simulink model "Intergration_simu"  (R2018b)
settings: Solver=FixedStepDiscrete  StartTime=0.0  StopTime=14  FixedStep=0.005  RelTol=1e-3
PostLoadFcn:
  | if any(exist('dsrtsu_mdlpostloadfcn', 'file') ~= 0), dsrtsu_mdlpostloadfcn('Execute', bdroot); end
values from neighbouring files (symbols this model uses):
  P_x165_On = 1.0    [CAN_Tx.sldd]
  P_x242_On = 1.0    [CAN_Tx.sldd]
  P_x246_On = 1.0    [CAN_Tx.sldd]
libraries: rtican x112, simulink x59
(part 25 of 31)

== system Intergration_simu/Radar410_RX/x80 ==
  Bus Creator1 : BusCreator  Inputs=11
  FRS_Status : rtican/RTICAN Receive (RX)   Reserved1=[]  Reserved2=[]  Reserved3=[]  Reserved4=[]  SfcnMessage=[]  Msg_Struct=[]  BoardTypeNo=[]  BoardNo=[]  ChannelNo=[]  Parameters=[]  DialogFcn=[]  UnitName=[]  Revision=[]  UnitValues=[]  DSProperties=struct('RTI',struct('Version',uint32(5),'BlockType',struct('isSLSource',uint8(1),'isSLSink',uint8(1),'isHWSource',uint8(0),'isHWSink',uint8(0),'isSetup',uint8(0),'isInline',uint8(1),'isNonInline',uint8(0),'isInterrupt',uint8(0),'isChannelwise',uint8(0)),'IOBoardType','RTICAN','UnitType','MESSAGE','Identifier','RX','DialogType','MSVC','BlockSet','RTICAN','SlaveProcessor','CAN'))  RTIBlockInterface=struct('OutputPortsWidth',int32([1 1 1 1 1 1 1 1 1 1 1 1 1 1]),'OutputPortsActive',ones(1,14),'OutputPortsName',{{'FRS_Msg_CheckSum','FRS_Msg_AliveCounter','FRS_Status_MisAlign','FRS_Status_HWErr','FRS_Status_BlkProg','FRS_Fail','FRS_MeasEnabled','FRS_Host_Yaw','FRS_HostSpeed','FRS_TimeStamp','FRS_Latency',['RX status'],['RX time'],['RX delta time']}},'OutputPortsDataType',{{'SS_DOUBLE','SS_DOUBLE','SS_DOUBLE','SS_DOUBLE','SS_DOUBLE','SS_DOUBLE','SS_DOUBLE','SS_DOUBLE','SS_DOUBLE','SS_DOUBLE','SS_DOUBLE','SS_DOUBLE','SS_DOUBLE','SS_DOUBLE'}},'OutputPortsLabel',{{'FRS_Msg_CheckSum','FRS_Msg_AliveCounter','FRS_Status_MisAlign','FRS_Status_HWErr','FRS_Status_BlkProg','FRS_Fail','FRS_MeasEnabled','FRS_Host_Yaw','FRS_HostSpeed','FRS_TimeStamp','FRS_Latency','','',''}},'OutputPortsLabelMode','ON','InputPortsWidth',int32(0),'InputPortsActive',0,'DialogFcn','rtican_message_interface_gui','BlockDisplay',{{'','center'}},'IconTransparency','on','ParameterTunableNames',{{}},'InitLevel',3,'BlockName',struct('Token',{{'FRS_Status'}}),'SampleTime',{{-1}},'TriggerPort',{{'none'}},'EnablePort',{{'none'}})  RTIBlockParameters="struct('BoardTypeNo',{{1,'OFF',[]}},'BoardNo',{{2,'ON',[1 16]}},'ChannelNo',{{2,'ON',[1 2]}},'Parameters',{{struct('DataFileSupport',struct('DataFileSelectedMaster',1,'DataFileSelectedLocal',1,'DataFileName','c:\\users\\linqi\\desktop\\matlab\\acc\\dbc\\ars410od_privatecan.dbc|','DataFileDate',{{{['24-11月-2020 15:06:17']}}},'SelectedFile','..\\..\\dbc\\ars410od_privatecan.dbc'),'Options',struct('StatusSelected',1,'TimeSelected',1,'DeltaTimeSelected',1,'BytePortSelected',0,'MessageLengthSelected',0,'TriggerPort',struct('Selected',0,'TriggerType',0),'UserCoding',struct('Selected',0,'InterfaceFile','UserDecodingFile','FcnName','UserDecodeFcn','InportSelected',0,'InportWidth',1,'OutportSelected',0,'OutportWidth',1),'EnablePortSelected',0,'SignalOnPortnameSelected',1,'UseRXService',0),'Message',struct('MsgOnBlocknameSelected',1,'MsgName','FRS_Status','MsgIdFormat',0,'MsgId',128,'MsgLength',8,'NumSignals',11,'SampleTime',-1,'Signal',struct('SgnName',{'FRS_Msg_CheckSum','FRS_Msg_AliveCounter','FRS_Status_MisAlign','FRS_Status_HWErr','FRS_Status_BlkProg','FRS_Fail','FRS_MeasEnabled','FRS_Host_Yaw','FRS_HostSpeed','FRS_TimeStamp','FRS_Latency'},'SgnStartBit',{0,8,12,15,16,17,18,19,30,42,58},'SgnLength',{8,4,3,1,1,1,1,11,12,16,6},'SgnType',{0,0,0,0,0,0,0,0,0,0,0},'ModeValue',{-1,-1,-1,-1,-1,-1,-1,-1,-1,-1,-1},'DataType',{0,0,0,0,0,0,0,0,0,0,0},'ByteLayout',{2,2,2,2,2,2,2,2,2,2,2},'Factor',{1,1,1,1,1,1,1,0.1,0.025,1,2},'Offset',{0,0,0,0,0,0,0,-102.4,-20,0,0},'SgnComment',{{['Check sum shall be generated out of each message content. check sum generation logic is TBC.']},{['Alive counter shall be incremented every radar sensor measurement cycle.']},{['This signal indicates radar sensor mis-alignment status.' char(10) '0x00:unknown' char(10) '0x01:calibrated' char(10) '0x02:sensor mis-alignment detected' char(10) '0x03:calibration in progress' char(10) '0x04:uncalibratable' char(10) '0x05-07:  reserved']},{['Flag to indicate if HW is failed or not.' char(10) '0x0:HW is NOT failed' char(10) '0x1:HW is failed']},{['Sensor blockage status indication.' char(10) '0x0: FRS is NOT blocked' char(10) '0x1: FRS is blocked']},{['This signal indicates if radar is working or not.' char(10) '0x0 = FRS radar is NOT working' char(10) '0x1 = FRS radar is working']},{['This signal indicates if the radar sensor is performing measurement or not. (radio-wave emission or not) Since Conti does not have this, it could be setup as the same as FRS_Fail.' char(10) '']},{['Host vehicle yaw rate in deg/s which is used for radar object tracking (calibrated host yaw rate if sensor has calibration capability).' char(10) 'Left turn is defined as FRS_Host_Yaw positive direction.']},{['Host vehicle over-ground speed which is used for radar object tracking (calibrated host velocity if the sensor has calibaration capability).' char(10) 'Forward movement is defined as FRS_HostSpeed positive direction.']},{['Sensor internal time stamp since the last sensor start up. the time stamp shall loop as it overflows.']},{['Radar process latency in ms from radio-wave reflection observation to CAN message transmission for current cycle.']}},'SgnUnit',{'n/a','n/a','n/a','n/a','n/a','','n/a','deg/s','m/s','s','ms'},'Min',{0,0,0,0,0,0,0,-102.4,-20,0,0},'Max',{255,15,7,1,1,1,1,102.3,82.375,65535,126},'SLDataType',{'SS_DOUBLE','SS_DOUBLE','SS_DOUBLE','SS_DOUBLE','SS_DOUBLE','SS_DOUBLE','SS_DOUBLE','SS_DOUBLE','SS_DOUBLE','SS_DOUBLE','SS_DOUBLE'}),'MsgIdNumFormat',0,'MsgComment',{{'FRS_Status'}}),'Version',1.2,'general',struct('isFromLib',0)),'OFF',[]}},'GroupId',{{struct('Group',{{'RTICAN'}},'No',2,'Behavior',{{'NAMECHANGE'}},'BlockType',{{'SINK'}},'NameChangeFlag',0),'OFF',[]}},'SFcnRTICANMessage',{{struct('MsgType','RX','SFcnPortType','Scalar','MsgName','FRS_Status','MsgIdFormat','STD','MsgId',128,'MsgLength',8,'NumSignals',11,'SampleTime',-1,'Signal',struct('SgnName',{'FRS_Msg_CheckSum','FRS_Msg_AliveCounter','FRS_Status_MisAlign','FRS_Status_HWErr','FRS_Status_BlkProg','FRS_Fail','FRS_MeasEnabled','FRS_Host_Yaw','FRS_HostSpeed','FRS_TimeStamp','FRS_Latency'},'SgnStartBit',{0,8,12,15,16,17,18,19,30,42,58},'SgnLength',{8,4,3,1,1,1,1,11,12,16,6},'SgnType',{'standard','standard','standard','standard','standard','standard','standard','standard','standard','standard','standard'},'ModeValue',{-1,-1,-1,-1,-1,-1,-1,-1,-1,-1,-1},'DataType',{['unsigned int'],['unsigned int'],['unsigned int'],['unsigned int'],['unsigned int'],['unsigned int'],['unsigned int'],['unsigned int'],['unsigned int'],['unsigned int'],['unsigned int']},'ByteLayout',{['motorola back.'],['motorola back.'],['motorola back.'],['motorola back.'],['motorola back.'],['motorola back.'],['motorola back.'],['motorola back.'],['motorola back.'],['motorola back.'],['motorola back.']},'Factor',{1,1,1,1,1,1,1,0.1,0.025,1,2},'Offset',{0,0,0,0,0,0,0,-102.4,-20,0,0},'SLDataType',{'SS_DOUBLE','SS_DOUBLE','SS_DOUBLE','SS_DOUBLE','SS_DOUBLE','SS_DOUBLE','SS_DOUBLE','SS_DOUBLE','SS_DOUBLE','SS_DOUBLE','SS_DOUBLE'}),'StatusSelected','yes','TimeSelected','yes','DeltaTimeSelected','yes','BytePortSelected','no','MessageLengthSelected','no','TriggerPort',struct('Selected','no','TriggerType',0),'UserCoding',struct('Selected','no','InterfaceFile','UserDecodingFile','FcnName','UserDecodeFcn','InportSelected','no','InportWidth',1,'OutportSelected','no','OutportWidth',1),'EnablePortSelected','no','UseRXService','no','BoardType','DS1','BoardNo',1,'ControllerNo',1),'OFF',[]}},'TLCFileName',{{'rtican_rx_message','OFF',[]}})"  RTISFcnParameters=struct('SFcnRTICANMessage','struct','TLCFileName','char')  RTIBlockParaDefault=struct('BoardTypeNo',4302,'BoardNo',1,'ChannelNo',1,'Parameters',struct('DataFileSupport',struct('DataFileSelectedMaster',0,'DataFileSelectedLocal',0,'DataFileName','','DataFileDate','','SelectedFile',['<no file selected>']),'Options',struct('StatusSelected',1,'TimeSelected',1,'DeltaTimeSelected',1,'BytePortSelected',0,'MessageLengthSelected',0,'TriggerPort',struct('Selected',0,'TriggerType','rising'),'UserCoding',struct('Selected',0,'InterfaceFile','UserDecodingFile','FcnName','UserDecodeFcn','InportSelected',0,'InportWidth',1,'OutportSelected',0,'OutportWidth',1),'EnablePortSelected',0,'SignalOnPortnameSelected',1,'UseRXService',0),'Message',struct('MsgOnBlocknameSelected',0,'MsgName',['RX Message'],'MsgIdFormat',0,'MsgId',100,'MsgLength',8,'NumSignals',1,'SampleTime',-1,'Signal',struct('SgnName',['RX signal'],'SgnStartBit',0,'SgnLength',8,'SgnType',0,'ModeValue',-1,'DataType',0,'SLDataType','SS_DOUBLE','ByteLayout',0,'Factor',1,'Offset',0,'Min',0,'Max',255,'SgnComment',{{}},'SgnUnit',''),'MsgIdNumFormat',0,'MsgComment',{{''}}),'Version',1.2,'general',struct('isFromLib',1)),'GroupId',struct('Group',{{'RTICAN'}},'No',1,'Behavior',{{'NAMECHANGE'}},'BlockType',{{'SINK'}},'NameChangeFlag',0),'SFcnRTICANMessage',struct('MsgType','RX','MsgName',['RX Message'],'MsgIdFormat','STD','MsgId',100,'MsgLength',8,'NumSignals',1,'SampleTime',-1,'Signal',struct('SgnName',['RX signal'],'SgnStartBit',0,'SgnLength',8,'SgnType','standard','ModeValue',-1,'DataType',['unsigned int'],'ByteLayout',['little endian'],'SLDataType','SS_DOUBLE','Factor',1,'Offset',0),'StatusSelected','yes','TimeSelected','yes','DeltaTimeSelected','yes','BytePortSelected','no','MessageLengthSelected','no','EnablePortSelected','no','UserCoding',struct('Selected','no','InterfaceFile','UserDecodingFile','FcnName','UserDecodeFcn','InportSelected','no','InportWidth',1,'OutportSelected','no','OutportWidth',1),'TriggerPort',struct('Selected','no','TriggerType','rising'),'UseRXService','no','BoardType','DS4302','BoardNo',1,'ControllerNo',1,'SFcnPortType','Scalar'),'TLCFileName','rtican_rx_message')
      settings: AttributesFormatString=Group Id: RTICAN2\n  SourceProductName=dSPACE RTI CAN Blockset
  Terminator : Terminator
  Terminator1 : Terminator
  Terminator2 : Terminator
  Out1 : Outport
  wires:
  FRS_Status/14 -> Terminator2/1
  FRS_Status/13 -> Terminator1/1
  FRS_Status/12 -> Terminator/1
  Bus Creator1/1 -> Out1/1
  FRS_Status/1 -> Bus Creator1/1  "FRS_Msg_CheckSum"
  FRS_Status/2 -> Bus Creator1/2  "FRS_Msg_AliveCounter"
  FRS_Status/3 -> Bus Creator1/3  "FRS_Status_MisAlign"
  FRS_Status/4 -> Bus Creator1/4  "FRS_Status_HWErr"
  FRS_Status/5 -> Bus Creator1/5  "FRS_Status_BlkProg"
  FRS_Status/6 -> Bus Creator1/6  "FRS_Fail"
  FRS_Status/7 -> Bus Creator1/7  "FRS_MeasEnabled"
  FRS_Status/8 -> Bus Creator1/8  "FRS_Host_Yaw"
  FRS_Status/9 -> Bus Creator1/9  "FRS_HostSpeed"
  FRS_Status/10 -> Bus Creator1/10  "FRS_TimeStamp"
  FRS_Status/11 -> Bus Creator1/11  "FRS_Latency"

== system Intergration_simu/TX/Adapter_Tx ==
  VLC_LgtCmd_st : Inport  OutDataTypeStr=Bus: VLC_LGTCMD_ST
  ACC_LgtCtrl_st : Inport  Port=2
  ATS_Po_st : Inport  Port=3
  Bus Selector : BusSelector  OutputSignals=Valid,dx,dy,Type
  Bus Selector1 : BusSelector  OutputSignals=ACCvSet
  Bus Selector4 : BusSelector  OutputSignals=EngineTorqReq,EngineTorqReqSt,ACCState,CDDEnable,CDDAxtar,CDDDriveoffReq,CDDStandstillReq
  calc_0x165 : Subsystem
  calc_0x242 : Subsystem
  calc_0x246 : Subsystem
  calc_0x255 : Subsystem
  x242 : Outport  OutDataTypeStr=Bus: x242
  x165 : Outport  Port=2  OutDataTypeStr=Bus: x165
  x246 : Outport  Port=3  OutDataTypeStr=Bus: x246
  x255 : Outport  Port=4  OutDataTypeStr=Bus: x255
  wires:
  VLC_LgtCmd_st/1 -> Bus Selector4/1  "VLC_LgtCmd_st"
  ATS_Po_st/1 -> Bus Selector/1
  ACC_LgtCtrl_st/1 -> Bus Selector1/1
  Bus Selector4/1 -> calc_0x165/1(<EngineTorqReq>)  "<EngineTorqReq>"
  Bus Selector4/2 -> calc_0x165/2(<EngineTorqReqSt>)  "<EngineTorqReqSt>"
  calc_0x165/1(COM_x165_st) -> x165/1
  Bus Selector4/3 -> calc_0x255/2(ACCState), calc_0x242/1(<ACCState>)  "<ACCState>"
  Bus Selector4/4 -> calc_0x242/2(<CDDEnable>)  "<CDDEnable>"
  Bus Selector4/5 -> calc_0x242/3(<CDDAxtar>)  "<CDDAxtar>"
  Bus Selector4/6 -> calc_0x242/4(<CDDDriveoffReq>)  "<CDDDriveoffReq>"
  Bus Selector4/7 -> calc_0x242/5(<CDDStandstillReq>)  "<CDDStandstillReq>"
  calc_0x242/1(COM_x242_st) -> x242/1
  Bus Selector/1 -> calc_0x246/1(<Valid>)  "<Valid>"
  Bus Selector/2 -> calc_0x255/3(dx), calc_0x246/2(<dx>)  "<dx>"
  Bus Selector1/1 -> calc_0x255/1(ACCvSet), calc_0x246/3(<ACCvSet>)  "<ACCvSet>"
  calc_0x246/1(Out1) -> x246/1
  calc_0x255/1(Out1) -> x255/1
  Bus Selector/4 -> calc_0x255/5(Type)  "<Type>"
  Bus Selector/3 -> calc_0x255/4(dy)  "<dy>"

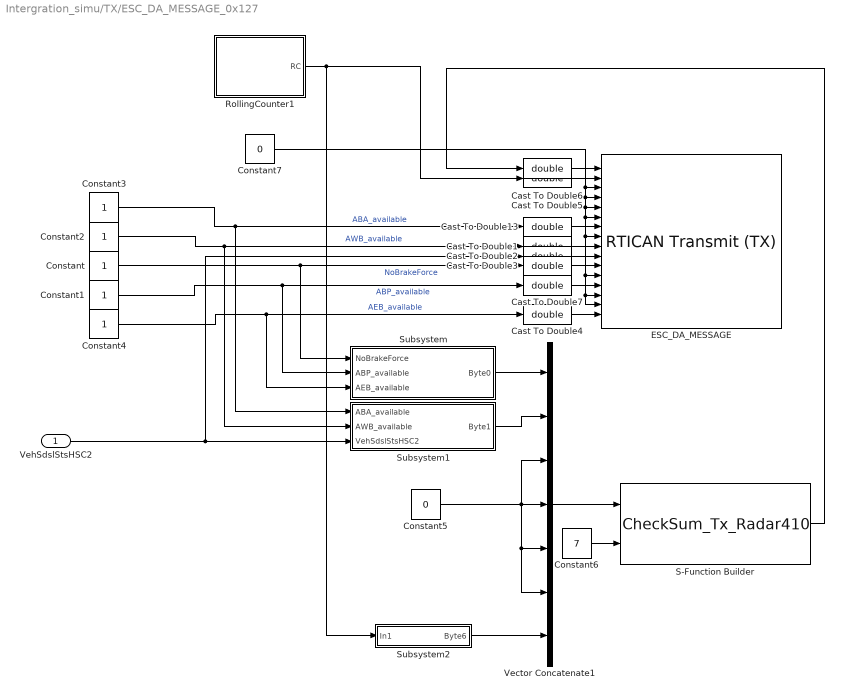
== system Intergration_simu/TX/ESC_DA_MESSAGE_0x127 ==
  VehSdslStsHSC2 : Inport
  Cast To Double{1..7,13} (8 alike) : DataTypeConversion  OutDataTypeStr=double
  Constant{,1..4} (5 alike) : Constant  OutDataTypeStr=single
  Constant5 : Constant  Value=0  OutDataTypeStr=uint8
  Constant6 : Constant  Value=7  OutDataTypeStr=uint8
  Constant7 : Constant  Value=0  OutDataTypeStr=double
  ESC_DA_MESSAGE : rtican/RTICAN Transmit (TX)   Reserved1=[]  Reserved2=[]  Reserved3=[]  Reserved4=[]  SfcnMessage=[]  Msg_Struct=[]  BoardTypeNo=[]  BoardNo=[]  ChannelNo=[]  Parameters=[]  DialogFcn=[]  UnitName=[]  Revision=[]  UnitValues=[]  DSProperties=struct('RTI',struct('Version',uint32(5),'BlockType',struct('isSLSource',uint8(1),'isSLSink',uint8(1),'isHWSource',uint8(0),'isHWSink',uint8(0),'isSetup',uint8(0),'isInline',uint8(1),'isNonInline',uint8(0),'isInterrupt',uint8(0),'isChannelwise',uint8(0)),'IOBoardType','RTICAN','UnitType','MESSAGE','Identifier','TX','DialogType','MSVC','BlockSet','RTICAN','SlaveProcessor','CAN'))  RTIBlockInterface=struct('InputPortsWidth',int32([1 1 1 1 1 1 1 1 1 1 1 1 1 1 1 1]),'InputPortsActive',ones(1,16),'InputPortsName',{{'ESC_DA_MESSAGE_Checksum','ESC_DA_MESSAGE_AliveCounter','ESC_DTC_Active','ESC_BrakeTempTooHigh','ESC_QDCFRS','ESC_ABA_active','ESC_ABA_available','ESC_AWB_active','ESC_AWB_available','ESC_Vehiclestandstill','ESC_NoBrakeForce','ESC_DiagExtModSts','ESC_ABP_available','ESC_ABP_active','ESC_AEB_active','ESC_AEB_available'}},'InputPortsDataType',{{'SS_DOUBLE','SS_DOUBLE','SS_DOUBLE','SS_DOUBLE','SS_DOUBLE','SS_DOUBLE','SS_DOUBLE','SS_DOUBLE','SS_DOUBLE','SS_DOUBLE','SS_DOUBLE','SS_DOUBLE','SS_DOUBLE','SS_DOUBLE','SS_DOUBLE','SS_DOUBLE'}},'OutputPortsWidth',int32([1 1 1 1]),'OutputPortsActive',[1 1 1 1],'OutputPortsName',{{['TX status'],['TX time'],['TX delta time'],['TX delay time']}},'DialogFcn','rtican_message_interface_gui','BlockDisplay',{{'','center'}},'IconTransparency','on','InitLevel',3,'BlockName',struct('Token',{{'ESC_DA_MESSAGE'}}),'SampleTime',{{-1}},'TriggerPort',{{'none'}},'EnablePort',{{'none'}})  RTIBlockParameters=struct('BoardTypeNo',{{1,'OFF',[]}},'BoardNo',{{3,'ON',[1 16]}},'ChannelNo',{{2,'ON',[1 2]}},'Parameters',{{struct('DataFileSupport',struct('DataFileSelectedMaster',1,'DataFileSelectedLocal',1,'DataFileName','c:\users\administrator.zx-201607042142\documents\matlab\zone\dbc\ars410od_privatecan.dbc|c:\users\administrator.zx-201607042142\desktop\zone\2020_demo\410\asr410od_public_can.dbc|','DataFileDate',{{{''},{''}}},'SelectedFile','..\..\..\..\..\desktop\zone\2020_demo\410\asr410od_public_can.dbc','InterfaceFcn','rtican_dbc_file_parser'),'Options',struct('StatusSelected',1,'TimeSelected',1,'DeltaTimeSelected',1,'DelayTimeSelected',1,'DelayTimeTXCommandSelected',0,'EncodeSetUnusedBitsToOne',0,'EnableMsgLoopback',0,'TriggerPort',struct('Selected',0,'TriggerType',0),'EnablePortSelected',0,'SignalOnPortnameSelected',1,'UserCoding',struct('Selected',0,'InterfaceFile','UserEncodingFile','FcnName','UserEncodeFcn','InportSelected',0,'InportWidth',1,'OutportSelected',0,'OutportWidth',1),'TerminationMsg',struct('Selected',0,'Byte0_7','0'),'InitialMsg',struct('Selected',0,'Byte0_7','0')),'Message',struct('MsgOnBlocknameSelected',1,'MsgName','ESC_DA_MESSAGE','MsgIdFormat',0,'MsgId',295,'MsgLength',8,'NumSignals',16,'SampleTime',-1,'StartTime',struct('Selected',0,'Value',3),'AutoRepeatTime',struct('Selected',0,'Value',0.1),'Timeout',struct('Selected',0,'Value',0.1),'DelayTime',struct('Selected',0,'Value',0.1),'Signal',struct('SgnName',{'ESC_DA_MESSAGE_Checksum','ESC_DA_MESSAGE_AliveCounter','ESC_DTC_Active','ESC_BrakeTempTooHigh','ESC_QDCFRS','ESC_ABA_active','ESC_ABA_available','ESC_AWB_active','ESC_AWB_available','ESC_Vehiclestandstill','ESC_NoBrakeForce','ESC_DiagExtModSts','ESC_ABP_available','ESC_ABP_active','ESC_AEB_active','ESC_AEB_available'},'SgnStartBit',{0,8,40,41,47,48,49,50,51,54,58,59,60,61,62,63},'SgnLength',{8,4,1,1,1,1,1,1,1,2,1,1,1,1,1,1},'SgnType',{0,0,0,0,0,0,0,0,0,0,0,0,0,0,0,0},'ModeValue',{-1,-1,-1,-1,-1,-1,-1,-1,-1,-1,-1,-1,-1,-1,-1,-1},'DataType',{0,0,0,0,0,0,0,0,0,0,0,0,0,0,0,0},'ByteLayout',{2,2,2,2,2,2,2,2,2,2,2,2,2,2,2,2},'Factor',{1,1,1,1,1,1,1,1,1,1,1,1,1,1,1,1},'Offset',{0,0,0,0,0,0,0,0,0,0,0,0,0,0,0,0},'SgnComment',{{'ESC_DA_MESSAGE_Checksum'},{'ESC_DA_MESSAGE_AliveCounter'},{'ESC_DTC_Active'},{'ESC_BrakeTempTooHigh'},{'ESC_QDCFRS'},{'ESC_ABA_active'},{'ESC_ABA_available'},{'ESC_AWB_active'},{'ESC_AWB_available'},{'ESC_Vehiclestandstill'},{'ESC_NoBrakeForce'},{'ESC_DiagExtModSts'},{'ESC_ABP_available'},{'ESC_ABP_active'},{'ESC_AEB_active'},{'ESC_AEB_available'}},'SgnUnit',{'','','','','','','','','','','','','','','',''},'Min',{0,0,0,0,0,0,0,0,0,0,0,0,0,0,0,0},'Max',{255,15,1,1,1,1,1,1,1,3,1,1,1,1,1,1},'SLDataType',{'SS_DOUBLE','SS_DOUBLE','SS_DOUBLE','SS_DOUBLE','SS_DOUBLE','SS_DOUBLE','SS_DOUBLE','SS_DOUBLE','SS_DOUBLE','SS_DOUBLE','SS_DOUBLE','SS_DOUBLE','SS_DOUBLE','SS_DOUBLE','SS_DOUBLE','SS_DOUBLE'}),'MsgIdNumFormat',1,'MsgComment',{{''}}),'Version',1.2,'general',struct('isFromLib',0)),'OFF',[]}},'GroupId',{{struct('Group',{{'RTICAN'}},'No',3,'Behavior',{{'NAMECHANGE'}},'BlockType',{{'SINK'}},'NameChangeFlag',0),'OFF',[]}},'SFcnRTICANMessage',{{struct('MsgType','TX','SFcnPortType','Scalar','MsgName','ESC_DA_MESSAGE','MsgIdFormat','STD','MsgId',295,'MsgLength',8,'NumSignals',16,'SampleTime',-1,'StartTime',struct('Selected','no','Value',3),'AutoRepeatTime',struct('Selected','no','Value',0.1),'Timeout',struct('Selected','no','Value',0.1),'Signal',struct('SgnName',{'ESC_DA_MESSAGE_Checksum','ESC_DA_MESSAGE_AliveCounter','ESC_DTC_Active','ESC_BrakeTempTooHigh','ESC_QDCFRS','ESC_ABA_active','ESC_ABA_available','ESC_AWB_active','ESC_AWB_available','ESC_Vehiclestandstill','ESC_NoBrakeForce','ESC_DiagExtModSts','ESC_ABP_available','ESC_ABP_active','ESC_AEB_active','ESC_AEB_available'},'SgnStartBit',{0,8,40,41,47,48,49,50,51,54,58,59,60,61,62,63},'SgnLength',{8,4,1,1,1,1,1,1,1,2,1,1,1,1,1,1},'SgnType',{'standard','standard','standard','standard','standard','standard','standard','standard','standard','standard','standard','standard','standard','standard','standard','standard'},'ModeValue',{-1,-1,-1,-1,-1,-1,-1,-1,-1,-1,-1,-1,-1,-1,-1,-1},'DataType',{['unsigned int'],['unsigned int'],['unsigned int'],['unsigned int'],['unsigned int'],['unsigned int'],['unsigned int'],['unsigned int'],['unsigned int'],['unsigned int'],['unsigned int'],['unsigned int'],['unsigned int'],['unsigned int'],['unsigned int'],['unsigned int']},'ByteLayout',{['motorola back.'],['motorola back.'],['motorola back.'],['motorola back.'],['motorola back.'],['motorola back.'],['motorola back.'],['motorola back.'],['motorola back.'],['motorola back.'],['motorola back.'],['motorola back.'],['motorola back.'],['motorola back.'],['motorola back.'],['motorola back.']},'Factor',{1,1,1,1,1,1,1,1,1,1,1,1,1,1,1,1},'Offset',{0,0,0,0,0,0,0,0,0,0,0,0,0,0,0,0},'SLDataType',{'SS_DOUBLE','SS_DOUBLE','SS_DOUBLE','SS_DOUBLE','SS_DOUBLE','SS_DOUBLE','SS_DOUBLE','SS_DOUBLE','SS_DOUBLE','SS_DOUBLE','SS_DOUBLE','SS_DOUBLE','SS_DOUBLE','SS_DOUBLE','SS_DOUBLE','SS_DOUBLE'}),'StatusSelected','yes','TimeSelected','yes','DeltaTimeSelected','yes','DelayTimeSelected','yes','DelayTimeTXCommandSelected','no','EncodeSetUnusedBitsToOne','no','EnableMsgLoopback','no','TriggerPort',struct('Selected','no','TriggerType',0),'EnablePortSelected','no','UserCoding',struct('Selected','no','InterfaceFile','UserEncodingFile','FcnName','UserEncodeFcn','InportSelected','no','InportWidth',1,'OutportSelected','no','OutportWidth',1),'TerminationMsg',struct('Selected','no','Byte0','0x00','Byte1','0x00','Byte2','0x00','Byte3','0x00','Byte4','0x00','Byte5','0x00','Byte6','0x00','Byte7','0x00'),'InitialMsg',struct('Selected','no','Byte0','0x00','Byte1','0x00','Byte2','0x00','Byte3','0x00','Byte4','0x00','Byte5','0x00','Byte6','0x00','Byte7','0x00'),'BoardType','DS1','BoardNo',3,'ControllerNo',2),'OFF',[]}},'TLCFileName',{{'rtican_tx_message','OFF',[]}})  RTISFcnParameters=struct('SFcnRTICANMessage','struct','TLCFileName','char')  RTIBlockParaDefault=struct('BoardTypeNo',4302,'BoardNo',1,'ChannelNo',1,'Parameters',struct('DataFileSupport',struct('DataFileSelectedMaster',0,'DataFileSelectedLocal',0,'DataFileName','','DataFileDate','','SelectedFile',['<no file selected>']),'Options',struct('StatusSelected',1,'TimeSelected',1,'DeltaTimeSelected',1,'DelayTimeSelected',1,'DelayTimeTXCommandSelected',0,'EncodeSetUnusedBitsToOne',0,'EnableMsgLoopback',0,'TriggerPort',struct('Selected',0,'TriggerType','rising'),'EnablePortSelected',0,'SignalOnPortnameSelected',1,'UserCoding',struct('Selected',0,'InterfaceFile','UserEncodingFile','FcnName','UserEncodeFcn','InportSelected',0,'InportWidth',1,'OutportSelected',0,'OutportWidth',1),'TerminationMsg',struct('Selected',0,'Byte0_7','0'),'InitialMsg',struct('Selected',0,'Byte0_7','0')),'Message',struct('MsgOnBlocknameSelected',0,'MsgName',['TX Message'],'MsgIdFormat',0,'MsgId',100,'MsgLength',8,'NumSignals',1,'SampleTime',-1,'StartTime',struct('Selected',0,'Value',0),'AutoRepeatTime',struct('Selected',0,'Value',0.1),'Timeout',struct('Selected',0,'Value',0.1),'DelayTime',struct('Selected',0,'Value',0.1),'Signal',struct('SgnName',['TX signal'],'SgnStartBit',0,'SgnLength',8,'SgnType',0,'ModeValue',-1,'DataType',0,'SLDataType','SS_DOUBLE','ByteLayout',0,'Factor',1,'Offset',0,'Min',0,'Max',255,'SgnComment',{{}},'SgnUnit',''),'MsgIdNumFormat',0,'MsgComment',{{''}}),'Version',1.2,'general',struct('isFromLib',1)),'GroupId',struct('Group',{{'RTICAN'}},'No',1,'Behavior',{{'NAMECHANGE'}},'BlockType',{{'SINK'}},'NameChangeFlag',0),'SFcnRTICANMessage',struct('MsgType','TX','MsgName',['TX Message'],'MsgIdFormat','STD','MsgId',100,'MsgLength',2,'NumSignals',1,'SampleTime',-1,'StartTime',struct('Selected','no','Value',0),'AutoRepeatTime',struct('Selected','no','Value',0.1),'Timeout',struct('Selected','no','Value',0.1),'DelayTime',struct('Selected','no','Value',0.1),'Signal',struct('SgnName',['TX signal'],'SgnStartBit',0,'SgnLength',8,'SgnType','standard','ModeValue',-1,'DataType',['unsigned int'],'ByteLayout',['little endian'],'SLDataType','SS_DOUBLE','Factor',1,'Offset',0),'StatusSelected','yes','TimeSelected','yes','DeltaTimeSelected','yes','DelayTimeSelected','yes','EnablePortSelected','no','EnableMsgLoopback','no','DelayTimeTXCommandSelected','no','EncodeSetUnusedBitsToOne','no','UserCoding',struct('Selected','no','InterfaceFile','UserDecodingFile','FcnName','UserDecodeFcn','InportSelected','no','InportWidth',1,'OutportSelected','no','OutportWidth',1),'TerminationMsg',struct('Selected','no','Byte0','0x00','Byte1','0x00','Byte2','0x00','Byte3','0x00','Byte4','0x00','Byte5','0x00','Byte6','0x00','Byte7','0x00'),'InitialMsg',struct('Selected','no','Byte0','0x00','Byte1','0x00','Byte2','0x00','Byte3','0x00','Byte4','0x00','Byte5','0x00','Byte6','0x00','Byte7','0x00'),'TriggerPort',struct('Selected','no','TriggerType','rising'),'BoardType','DS4302','BoardNo',1,'ControllerNo',1,'SFcnPortType','Scalar'),'TLCFileName','rtican_tx_message')
      settings: AttributesFormatString=Group Id: RTICAN3\n  SourceProductName=dSPACE RTI CAN Blockset
  RollingCounter1 : Subsystem
  S-Function Builder : S-Function  InitFcn=try, set_param(gcb,'FunctionName','CheckSum_Tx_Radar410'), end  FunctionName=CheckSum_Tx_Radar410  SFunctionModules=CheckSum_Tx_Radar410_wrapper  SFunctionDeploymentMode=off  EnableBusSupport=off  mask(S-Function Builder){}
      mask help: Simulink:masks:SFunctionBuilder_MD
      mask init: same as Intergration_simu/Tx_410_10ms/S-Function Builder1
      settings: CopyFcn=set_param(gcbh,'LinkStatus','none')  PreSaveFcn=try, set_param(gcb,'FunctionName','CheckSum_Tx_Radar410'), end  OpenFcn=sfunctionwizard(gcbh)
      mask Display: plot(val(:,1),val(:,2)),disp(sys), port_label('input',1,'data'), port_label('input',2,'length'), port_label('output',1,'u8_crc8')
  Subsystem : Subsystem
  Subsystem1 : Subsystem
  Subsystem2 : Subsystem
  Vector Concatenate1 : Concatenate  NumInputs=7
  wires:
  RollingCounter1/1(RC) -> Subsystem2/1(In1), Cast To Double5/1
  Subsystem2/1(Byte6) -> Vector Concatenate1/7
  Subsystem/1(Byte0) -> Vector Concatenate1/1
  Constant2/1 -> Subsystem1/2(AWB_available), Cast To Double1/1  "AWB_available"
  Constant5/1 -> Vector Concatenate1/3, Vector Concatenate1/6, Vector Concatenate1/5, Vector Concatenate1/4
  Constant3/1 -> Subsystem1/1(ABA_available), Cast To Double13/1  "ABA_available"
  Vector Concatenate1/1 -> S-Function Builder/1
  Constant4/1 -> Subsystem/3(AEB_available), Cast To Double4/1  "AEB_available"
  Constant7/1 -> ESC_DA_MESSAGE/15, ESC_DA_MESSAGE/14, ESC_DA_MESSAGE/12, ESC_DA_MESSAGE/8, ESC_DA_MESSAGE/6, ESC_DA_MESSAGE/5, ESC_DA_MESSAGE/4, ESC_DA_MESSAGE/3
  Constant6/1 -> S-Function Builder/2
  Constant/1 -> Cast To Double3/1, Subsystem/1(NoBrakeForce)  "NoBrakeForce"
  Constant1/1 -> Cast To Double7/1, Subsystem/2(ABP_available)  "ABP_available"
  Cast To Double6/1 -> ESC_DA_MESSAGE/1
  Cast To Double4/1 -> ESC_DA_MESSAGE/16
  Subsystem1/1(Byte1) -> Vector Concatenate1/2
  Cast To Double3/1 -> ESC_DA_MESSAGE/11
  Cast To Double5/1 -> ESC_DA_MESSAGE/2
  VehSdslStsHSC2/1 -> Cast To Double2/1, Subsystem1/3(VehSdslStsHSC2)
  S-Function Builder/1 -> Cast To Double6/1
  Cast To Double13/1 -> ESC_DA_MESSAGE/7
  Cast To Double1/1 -> ESC_DA_MESSAGE/9
  Cast To Double2/1 -> ESC_DA_MESSAGE/10
  Cast To Double7/1 -> ESC_DA_MESSAGE/13

== system Intergration_simu/TX/ESC_FrontWheelSpeedKPH_0x123 ==
  <WhlGndVelLDrvn_Radar> : Inport
  <WhlGndVelRDrvn_Radar> : Inport  Port=2
  <LDrvnWhlRotlDircn> : Inport  Port=3
  <RDrvnWhlRotlDircn> : Inport  Port=4
  Cast To Double{1..6} (6 alike) : DataTypeConversion  OutDataTypeStr=double
  Constant : Constant  Value=0  OutDataTypeStr=uint8
  Constant1 : Constant  Value=0  OutDataTypeStr=double
  Constant6 : Constant  Value=7  OutDataTypeStr=uint8
  ESC_FrontWheelSpeedKPH : rtican/RTICAN Transmit (TX)   Reserved1=[]  Reserved2=[]  Reserved3=[]  Reserved4=[]  SfcnMessage=[]  Msg_Struct=[]  BoardTypeNo=[]  BoardNo=[]  ChannelNo=[]  Parameters=[]  DialogFcn=[]  UnitName=[]  Revision=[]  UnitValues=[]  DSProperties=struct('RTI',struct('Version',uint32(5),'BlockType',struct('isSLSource',uint8(1),'isSLSink',uint8(1),'isHWSource',uint8(0),'isHWSink',uint8(0),'isSetup',uint8(0),'isInline',uint8(1),'isNonInline',uint8(0),'isInterrupt',uint8(0),'isChannelwise',uint8(0)),'IOBoardType','RTICAN','UnitType','MESSAGE','Identifier','TX','DialogType','MSVC','BlockSet','RTICAN','SlaveProcessor','CAN'))  RTIBlockInterface=struct('InputPortsWidth',int32([1 1 1 1 1 1 1 1 1 1]),'InputPortsActive',[1 1 1 1 1 1 1 1 1 1],'InputPortsName',{{'ESC_FrontWheelSpeedsKPH_Checksum','ESC_FrontWheelSpeedsKPH_AliveCou','ESC_Mcylinder_PressureInvalid','ESC_Mcylinder_Pressure','ESC_FRWheelSpeedInvalid','ESC_FRWheelDirection','ESC_FRWheelSpeedKPH','ESC_FLWheelSpeedInvalid','ESC_FLWheelDirection','ESC_FLWheelSpeedKPH'}},'InputPortsDataType',{{'SS_DOUBLE','SS_DOUBLE','SS_DOUBLE','SS_DOUBLE','SS_DOUBLE','SS_DOUBLE','SS_DOUBLE','SS_DOUBLE','SS_DOUBLE','SS_DOUBLE'}},'OutputPortsWidth',int32([1 1 1 1]),'OutputPortsActive',[1 1 1 1],'OutputPortsName',{{['TX status'],['TX time'],['TX delta time'],['TX delay time']}},'DialogFcn','rtican_message_interface_gui','BlockDisplay',{{'','center'}},'IconTransparency','on','InitLevel',3,'BlockName',struct('Token',{{'ESC_FrontWheelSpeedKPH'}}),'SampleTime',{{-1}},'TriggerPort',{{'none'}},'EnablePort',{{'none'}})  RTIBlockParameters=struct('BoardTypeNo',{{1,'OFF',[]}},'BoardNo',{{3,'ON',[1 16]}},'ChannelNo',{{2,'ON',[1 2]}},'Parameters',{{struct('DataFileSupport',struct('DataFileSelectedMaster',1,'DataFileSelectedLocal',1,'DataFileName','c:\users\administrator.zx-201607042142\documents\matlab\zone\dbc\ars410od_privatecan.dbc|c:\users\administrator.zx-201607042142\desktop\zone\2020_demo\410\asr410od_public_can.dbc|','DataFileDate',{{{''},{['30-十一月-2020 09:38:41']}}},'SelectedFile','..\..\..\..\..\desktop\zone\2020_demo\410\asr410od_public_can.dbc','InterfaceFcn','rtican_dbc_file_parser'),'Options',struct('StatusSelected',1,'TimeSelected',1,'DeltaTimeSelected',1,'DelayTimeSelected',1,'DelayTimeTXCommandSelected',0,'EncodeSetUnusedBitsToOne',0,'EnableMsgLoopback',0,'TriggerPort',struct('Selected',0,'TriggerType',0),'EnablePortSelected',0,'SignalOnPortnameSelected',1,'UserCoding',struct('Selected',0,'InterfaceFile','UserEncodingFile','FcnName','UserEncodeFcn','InportSelected',0,'InportWidth',1,'OutportSelected',0,'OutportWidth',1),'TerminationMsg',struct('Selected',0,'Byte0_7','0'),'InitialMsg',struct('Selected',0,'Byte0_7','0')),'Message',struct('MsgOnBlocknameSelected',1,'MsgName','ESC_FrontWheelSpeedKPH','MsgIdFormat',0,'MsgId',291,'MsgLength',8,'NumSignals',10,'SampleTime',-1,'StartTime',struct('Selected',0,'Value',3),'AutoRepeatTime',struct('Selected',0,'Value',0.1),'Timeout',struct('Selected',0,'Value',0.1),'DelayTime',struct('Selected',0,'Value',0.1),'Signal',struct('SgnName',{'ESC_FrontWheelSpeedsKPH_Checksum','ESC_FrontWheelSpeedsKPH_AliveCou','ESC_Mcylinder_PressureInvalid','ESC_Mcylinder_Pressure','ESC_FRWheelSpeedInvalid','ESC_FRWheelDirection','ESC_FRWheelSpeedKPH','ESC_FLWheelSpeedInvalid','ESC_FLWheelDirection','ESC_FLWheelSpeedKPH'},'SgnStartBit',{0,8,12,24,32,33,35,48,49,51},'SgnLength',{8,4,1,8,1,2,13,1,2,13},'SgnType',{0,0,0,0,0,0,0,0,0,0},'ModeValue',{-1,-1,-1,-1,-1,-1,-1,-1,-1,-1},'DataType',{0,0,0,0,0,0,0,0,0,0},'ByteLayout',{2,2,2,2,2,2,2,2,2,2},'Factor',{1,1,1,1,1,1,0.05625,1,1,0.05625},'Offset',{0,0,0,0,0,0,0,0,0,0},'SgnComment',{{'ESC_FrontWheelSpeedsKPH_Checksum'},{'ESC_FrontWheelSpeedsKPH_AliveCou'},{'ESC_Mcylinder_PressureInvalid'},{'ESC_Mcylinder_Pressure'},{'ESC_FRWheelSpeedInvalid'},{'ESC_FRWheelDirection'},{'ESC_FRWheelSpeedKPH'},{'ESC_FLWheelSpeedInvalid'},{'ESC_FLWheelDirection'},{'ESC_FLWheelSpeedKPH'}},'SgnUnit',{'','','','','','','','','',''},'Min',{0,0,0,0,0,0,0,0,0,0},'Max',{255,15,1,254,1,3,460.6875,1,3,460.6875},'SLDataType',{'SS_DOUBLE','SS_DOUBLE','SS_DOUBLE','SS_DOUBLE','SS_DOUBLE','SS_DOUBLE','SS_DOUBLE','SS_DOUBLE','SS_DOUBLE','SS_DOUBLE'}),'MsgIdNumFormat',1,'MsgComment',{{''}}),'Version',1.2,'general',struct('isFromLib',0)),'OFF',[]}},'GroupId',{{struct('Group',{{'RTICAN'}},'No',3,'Behavior',{{'NAMECHANGE'}},'BlockType',{{'SINK'}},'NameChangeFlag',0),'OFF',[]}},'SFcnRTICANMessage',{{struct('MsgType','TX','SFcnPortType','Scalar','MsgName','ESC_FrontWheelSpeedKPH','MsgIdFormat','STD','MsgId',291,'MsgLength',8,'NumSignals',10,'SampleTime',-1,'StartTime',struct('Selected','no','Value',3),'AutoRepeatTime',struct('Selected','no','Value',0.1),'Timeout',struct('Selected','no','Value',0.1),'Signal',struct('SgnName',{'ESC_FrontWheelSpeedsKPH_Checksum','ESC_FrontWheelSpeedsKPH_AliveCou','ESC_Mcylinder_PressureInvalid','ESC_Mcylinder_Pressure','ESC_FRWheelSpeedInvalid','ESC_FRWheelDirection','ESC_FRWheelSpeedKPH','ESC_FLWheelSpeedInvalid','ESC_FLWheelDirection','ESC_FLWheelSpeedKPH'},'SgnStartBit',{0,8,12,24,32,33,35,48,49,51},'SgnLength',{8,4,1,8,1,2,13,1,2,13},'SgnType',{'standard','standard','standard','standard','standard','standard','standard','standard','standard','standard'},'ModeValue',{-1,-1,-1,-1,-1,-1,-1,-1,-1,-1},'DataType',{['unsigned int'],['unsigned int'],['unsigned int'],['unsigned int'],['unsigned int'],['unsigned int'],['unsigned int'],['unsigned int'],['unsigned int'],['unsigned int']},'ByteLayout',{['motorola back.'],['motorola back.'],['motorola back.'],['motorola back.'],['motorola back.'],['motorola back.'],['motorola back.'],['motorola back.'],['motorola back.'],['motorola back.']},'Factor',{1,1,1,1,1,1,0.05625,1,1,0.05625},'Offset',{0,0,0,0,0,0,0,0,0,0},'SLDataType',{'SS_DOUBLE','SS_DOUBLE','SS_DOUBLE','SS_DOUBLE','SS_DOUBLE','SS_DOUBLE','SS_DOUBLE','SS_DOUBLE','SS_DOUBLE','SS_DOUBLE'}),'StatusSelected','yes','TimeSelected','yes','DeltaTimeSelected','yes','DelayTimeSelected','yes','DelayTimeTXCommandSelected','no','EncodeSetUnusedBitsToOne','no','EnableMsgLoopback','no','TriggerPort',struct('Selected','no','TriggerType',0),'EnablePortSelected','no','UserCoding',struct('Selected','no','InterfaceFile','UserEncodingFile','FcnName','UserEncodeFcn','InportSelected','no','InportWidth',1,'OutportSelected','no','OutportWidth',1),'TerminationMsg',struct('Selected','no','Byte0','0x00','Byte1','0x00','Byte2','0x00','Byte3','0x00','Byte4','0x00','Byte5','0x00','Byte6','0x00','Byte7','0x00'),'InitialMsg',struct('Selected','no','Byte0','0x00','Byte1','0x00','Byte2','0x00','Byte3','0x00','Byte4','0x00','Byte5','0x00','Byte6','0x00','Byte7','0x00'),'BoardType','DS1','BoardNo',3,'ControllerNo',2),'OFF',[]}},'TLCFileName',{{'rtican_tx_message','OFF',[]}})  RTISFcnParameters=struct('SFcnRTICANMessage','struct','TLCFileName','char')  RTIBlockParaDefault=struct('BoardTypeNo',4302,'BoardNo',1,'ChannelNo',1,'Parameters',struct('DataFileSupport',struct('DataFileSelectedMaster',0,'DataFileSelectedLocal',0,'DataFileName','','DataFileDate','','SelectedFile',['<no file selected>']),'Options',struct('StatusSelected',1,'TimeSelected',1,'DeltaTimeSelected',1,'DelayTimeSelected',1,'DelayTimeTXCommandSelected',0,'EncodeSetUnusedBitsToOne',0,'EnableMsgLoopback',0,'TriggerPort',struct('Selected',0,'TriggerType','rising'),'EnablePortSelected',0,'SignalOnPortnameSelected',1,'UserCoding',struct('Selected',0,'InterfaceFile','UserEncodingFile','FcnName','UserEncodeFcn','InportSelected',0,'InportWidth',1,'OutportSelected',0,'OutportWidth',1),'TerminationMsg',struct('Selected',0,'Byte0_7','0'),'InitialMsg',struct('Selected',0,'Byte0_7','0')),'Message',struct('MsgOnBlocknameSelected',0,'MsgName',['TX Message'],'MsgIdFormat',0,'MsgId',100,'MsgLength',8,'NumSignals',1,'SampleTime',-1,'StartTime',struct('Selected',0,'Value',0),'AutoRepeatTime',struct('Selected',0,'Value',0.1),'Timeout',struct('Selected',0,'Value',0.1),'DelayTime',struct('Selected',0,'Value',0.1),'Signal',struct('SgnName',['TX signal'],'SgnStartBit',0,'SgnLength',8,'SgnType',0,'ModeValue',-1,'DataType',0,'SLDataType','SS_DOUBLE','ByteLayout',0,'Factor',1,'Offset',0,'Min',0,'Max',255,'SgnComment',{{}},'SgnUnit',''),'MsgIdNumFormat',0,'MsgComment',{{''}}),'Version',1.2,'general',struct('isFromLib',1)),'GroupId',struct('Group',{{'RTICAN'}},'No',1,'Behavior',{{'NAMECHANGE'}},'BlockType',{{'SINK'}},'NameChangeFlag',0),'SFcnRTICANMessage',struct('MsgType','TX','MsgName',['TX Message'],'MsgIdFormat','STD','MsgId',100,'MsgLength',2,'NumSignals',1,'SampleTime',-1,'StartTime',struct('Selected','no','Value',0),'AutoRepeatTime',struct('Selected','no','Value',0.1),'Timeout',struct('Selected','no','Value',0.1),'DelayTime',struct('Selected','no','Value',0.1),'Signal',struct('SgnName',['TX signal'],'SgnStartBit',0,'SgnLength',8,'SgnType','standard','ModeValue',-1,'DataType',['unsigned int'],'ByteLayout',['little endian'],'SLDataType','SS_DOUBLE','Factor',1,'Offset',0),'StatusSelected','yes','TimeSelected','yes','DeltaTimeSelected','yes','DelayTimeSelected','yes','EnablePortSelected','no','EnableMsgLoopback','no','DelayTimeTXCommandSelected','no','EncodeSetUnusedBitsToOne','no','UserCoding',struct('Selected','no','InterfaceFile','UserDecodingFile','FcnName','UserDecodeFcn','InportSelected','no','InportWidth',1,'OutportSelected','no','OutportWidth',1),'TerminationMsg',struct('Selected','no','Byte0','0x00','Byte1','0x00','Byte2','0x00','Byte3','0x00','Byte4','0x00','Byte5','0x00','Byte6','0x00','Byte7','0x00'),'InitialMsg',struct('Selected','no','Byte0','0x00','Byte1','0x00','Byte2','0x00','Byte3','0x00','Byte4','0x00','Byte5','0x00','Byte6','0x00','Byte7','0x00'),'TriggerPort',struct('Selected','no','TriggerType','rising'),'BoardType','DS4302','BoardNo',1,'ControllerNo',1,'SFcnPortType','Scalar'),'TLCFileName','rtican_tx_message')
      settings: AttributesFormatString=Group Id: RTICAN3\n  SourceProductName=dSPACE RTI CAN Blockset
  RollingCounter1 : Subsystem
  S-Function Builder1 : S-Function  InitFcn=try, set_param(gcb,'FunctionName','CheckSum_Tx_Radar410'), end  FunctionName=CheckSum_Tx_Radar410  SFunctionModules=CheckSum_Tx_Radar410_wrapper  SFunctionDeploymentMode=off  EnableBusSupport=off  mask(S-Function Builder){}
      mask help: Simulink:masks:SFunctionBuilder_MD
      mask init: same as Intergration_simu/Tx_410_10ms/S-Function Builder1
      settings: CopyFcn=set_param(gcbh,'LinkStatus','none')  PreSaveFcn=try, set_param(gcb,'FunctionName','CheckSum_Tx_Radar410'), end  OpenFcn=sfunctionwizard(gcbh)
      mask Display: plot(val(:,1),val(:,2)),disp(sys), port_label('input',1,'data'), port_label('input',2,'length'), port_label('output',1,'u8_crc8')
  Subsystem : Subsystem
  Subsystem1 : Subsystem
  Subsystem2 : Subsystem
  Subsystem3 : Subsystem
  Subsystem4 : Subsystem
  Vector Concatenate1 : Concatenate  NumInputs=7
  wires:
  Subsystem2/1(Out1) -> Cast To Double1/1
  <LDrvnWhlRotlDircn>/1 -> Cast To Double2/1, Subsystem1/2(<LDrvnWhlRotlDircn>)
  Subsystem4/1(Byte6) -> Vector Concatenate1/7
  Cast To Double1/1 -> ESC_FrontWheelSpeedKPH/7
  Constant1/1 -> ESC_FrontWheelSpeedKPH/3, ESC_FrontWheelSpeedKPH/8, ESC_FrontWheelSpeedKPH/5, ESC_FrontWheelSpeedKPH/4
  Vector Concatenate1/1 -> S-Function Builder1/1
  <WhlGndVelRDrvn_Radar>/1 -> Subsystem2/1(<WhlGndVelLDrvn_Radar>)
  <RDrvnWhlRotlDircn>/1 -> Cast To Double4/1, Subsystem3/2(<LDrvnWhlRotlDircn>)
  Cast To Double6/1 -> ESC_FrontWheelSpeedKPH/1
  Subsystem/3(Output) -> Subsystem1/1(In1)
  Subsystem2/3(Output) -> Subsystem3/1(In1)
  Subsystem2/2(Byte2) -> Vector Concatenate1/3
  RollingCounter1/1(RC) -> Cast To Double5/1, Subsystem4/1(In1)
  <WhlGndVelLDrvn_Radar>/1 -> Subsystem/1(<WhlGndVelLDrvn_Radar>)
  Subsystem1/1(Byte1) -> Vector Concatenate1/2
  Constant/1 -> Vector Concatenate1/6, Vector Concatenate1/5
  Cast To Double3/1 -> ESC_FrontWheelSpeedKPH/10
  Constant6/1 -> S-Function Builder1/2
  Cast To Double4/1 -> ESC_FrontWheelSpeedKPH/6
  Cast To Double2/1 -> ESC_FrontWheelSpeedKPH/9
  S-Function Builder1/1 -> Cast To Double6/1
  Subsystem/2(Byte0) -> Vector Concatenate1/1
  Subsystem3/1(Byte3) -> Vector Concatenate1/4
  Cast To Double5/1 -> ESC_FrontWheelSpeedKPH/2
  Subsystem/1(Out1) -> Cast To Double3/1
